simulink model "ControlSystem"  (R2025b)
settings: Solver=VariableStepAuto  StartTime=0.0  StopTime=5  RelTol=1e-3
libraries: simulink x1, simulink_extras x1
settings Model: Creator=Ranvir  LastModifiedBy=Ranvir

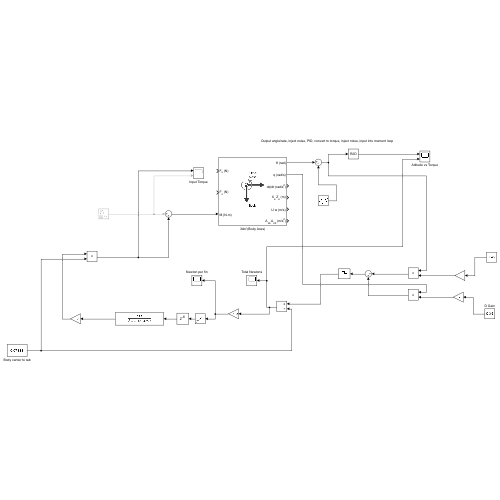
[thumbnail: Simulink's stored preview of the top-level diagram]
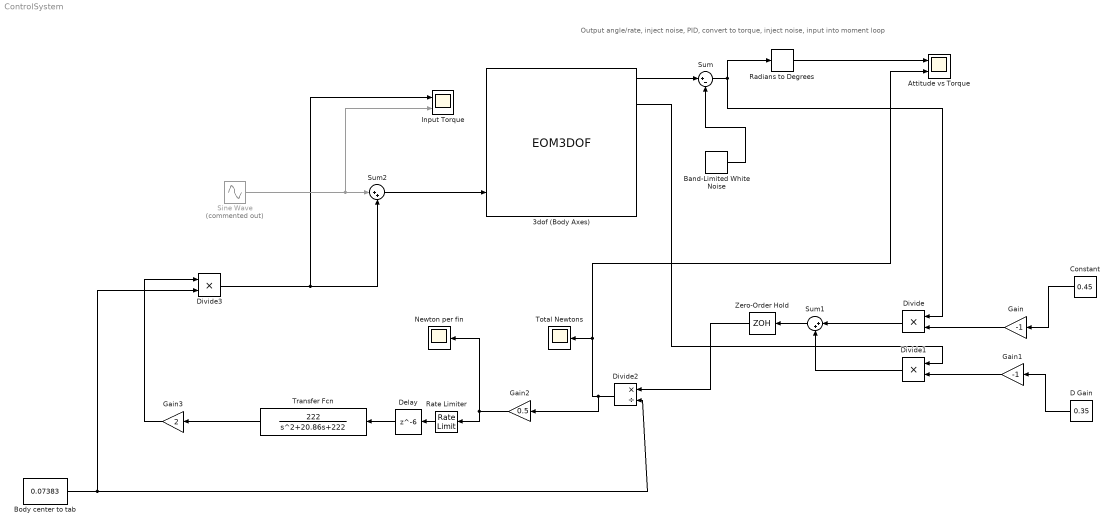
== system ControlSystem ==
  note: Output angle/rate, inject noise, PID, convert to torque, inject noise, input into moment loop
  3dof (Body Axes) : EOM3DOF  v_ini=0  theta_ini=deg2rad(30)  q_ini=0 %deg2rad(360)  mass=16.5  Iyy=0.14158  g=0
  Attitude vs Torque : Scope  NumInputPorts=2
      settings: ActiveDisplayYMinimum=-6.7048973098271221  ActiveDisplayYMaximum=35.28411457769829
  Band-Limited White Noise : simulink/Sources/Band-Limited White Noise  Cov=[1e-6]  Ts=0.01  seed=[23341]
  Body center to tab : Constant  Value=0.07383
  Constant : Constant  Value=0.45
  D Gain : Constant  Value=0.35
  Delay : Delay  DelayLength=6
  Divide : Product  Inputs=**
  Divide1 : Product  Inputs=**
  Divide2 : Product  Inputs=*/
  Divide3 : Product  Inputs=**
  Gain : Gain  Gain=-1
  Gain1 : Gain  Gain=-1
  Gain2 : Gain  Gain=0.5
  Gain3 : Gain  Gain=2
  Input Torque : Scope  NumInputPorts=2
      settings: ActiveDisplayYMinimum=-1  ActiveDisplayYMaximum=1  DataLoggingVariableName=ScopeData3
  Newton per fin : Scope
      settings: DataLoggingVariableName=ScopeData2
  Radians to Degrees : simulink_extras/Transformations/Radians to Degrees
  Rate Limiter : RateLimiter  RisingSlewLimit=61.6  FallingSlewLimit=-61.6  SampleTimeMode=inherited
  Sine Wave : Sin  Commented=on  SampleTime=0
  Sum : Sum  Inputs=|+-
  Sum1 : Sum  Inputs=|++
  Sum2 : Sum  Inputs=|++
  Total Newtons : Scope
      settings: ActiveDisplayYMinimum=-3.78412512894862  ActiveDisplayYMaximum=1.6209084704170538
  Transfer Fcn : TransferFcn  Numerator=[222]  Denominator=[1 20.86 222]
  Zero-Order Hold : ZeroOrderHold  SampleTime=0.002
  wires:
  Radians to Degrees/1 -> Attitude vs Torque/1
  Constant/1 -> Gain/1
  Gain/1 -> Divide/2
  D Gain/1 -> Gain1/1
  Gain1/1 -> Divide1/2
  3dof (Body Axes)/2 -> Divide1/1
  Divide/1 -> Sum1/1
  Divide1/1 -> Sum1/2
  Sum1/1 -> Zero-Order Hold/1
  Zero-Order Hold/1 -> Divide2/1
  Body center to tab/1 -> Divide3/2, Divide2/2
  Divide2/1 -> Gain2/1, Attitude vs Torque/2, Total Newtons/1
  Gain2/1 -> Newton per fin/1, Rate Limiter/1
  Delay/1 -> Transfer Fcn/1
  Transfer Fcn/1 -> Gain3/1
  Gain3/1 -> Divide3/1
  Sum2/1 -> 3dof (Body Axes)/3
  Divide3/1 -> Input Torque/1, Sum2/2
  Sine Wave/1 -> Input Torque/2, Sum2/1
  Rate Limiter/1 -> Delay/1
  Sum/1 -> Divide/1, Radians to Degrees/1
  3dof (Body Axes)/1 -> Sum/1
  Band-Limited White Noise/1 -> Sum/2
